simulink model "Design_qrate"  (R2017a)
settings: Solver=VariableStepAuto  StartTime=0.0  StopTime=20  RelTol=1e-3  EnableMultiTasking=on
InitFcn:
  | clear all; load('Parameters.mat');
undefined symbols (not defined in the file or in its folder): trim_control_hi
libraries: simulink x1
settings Model: Creator=Y Nie  LastModifiedBy=aelabuser
settings DataIOCC: SaveFormat=Array  SignalLoggingSaveFormat=ModelDataLogs  SaveOutput=off  SignalLogging=off  DSMLogging=off  TimeSaveName=DesignTime
settings OptimizationCC: ExpressionDepthLimit=2147483647  LifeSpan=inf
settings DebuggingCC: UnderspecifiedInitializationDetection=Classic  MergeDetectMultiDrivingBlocksExec=none  FcnCallInpInsideContextMsg=warning  StateNameClashWarn=warning  SFUnexpectedBacktrackingDiag=warning  SFNoUnconditionalDefaultTransitionDiag=warning  SFExecutionAtInitializationDiag=none
settings HardwareCC: ProdBitPerPointer=32  ProdBitPerSizeT=32  ProdBitPerPtrDiffT=32  ProdLargestAtomicFloat=None  ProdIntDivRoundTo=Undefined  ProdEndianess=Unspecified  ProdWordSize=32  ProdHWDeviceType=32-bit Generic
settings ModelReferenceCC: PropagateSignalLabelsOutOfModel=off
settings GRTTargetCC: TargetLangStandard=C89/C90 (ANSI)  GeneratePreprocessorConditionals=Disable all  CombineOutputUpdateFcns=off  GRTInterface=on
settings ConfigComp: CovMetricSettings=dw  CovHtmlReporting=on  CovSaveCumulativeToWorkspaceVar=on  CovSaveSingleToWorkspaceVar=on  CovExternalEMLEnable=off

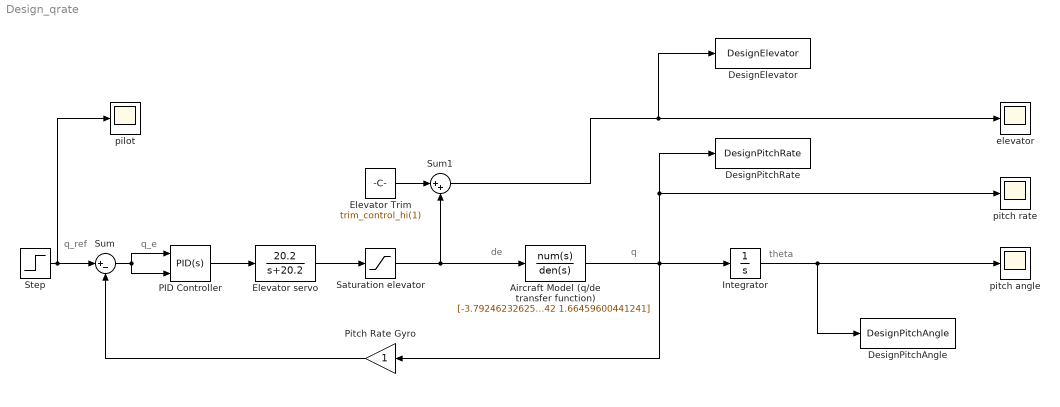
== system Design_qrate ==
  note: q_e
  note: de
  note: q
  note: theta
  note: q_ref
  Aircraft Model (q/de transfer function) : TransferFcn  Numerator=[-3.79246232625222 -2.17961147447550]  Denominator=[1 1.49753537373142 1.66459600441241]
  DesignElevator : ToWorkspace  VariableName=DesignElevator  SampleTime=-1
  DesignPitchAngle : ToWorkspace  VariableName=DesignPitchAngle  SampleTime=-1
  DesignPitchRate : ToWorkspace  VariableName=DesignPitchRate  SampleTime=-1
  Elevator Trim : Constant  Value=trim_control_hi(1)
  Elevator servo : TransferFcn  Numerator=[20.2]  Denominator=[1 20.2]
  Integrator : Integrator
  PID Controller : simulink/Continuous/PID Controller  Controller=PID  TimeDomain=Continuous-time  SampleTime=-1  IntegratorMethod=Forward Euler  FilterMethod=Forward Euler  Form=Parallel  UseFilter=on  ControllerParametersSource=internal  P=-10  I=-7  D=0  N=100  InitialConditionSource=internal  InitialConditionForIntegrator=0  InitialConditionForFilter=0  ExternalReset=either  LimitOutput=off  UpperSaturationLimit=inf  LowerSaturationLimit=-inf  LinearizeAsGain=on  AntiWindupMode=none  Kb=1  TrackingMode=off  Kt=1  PParamMin=[]  PParamMax=[]  IParamMin=[]  IParamMax=[]  DParamMin=[]  DParamMax=[]  NParamMin=[]  NParamMax=[]  KbParamMin=[]  KbParamMax=[]  KtParamMin=[]  KtParamMax=[]  POutMin=[]  POutMax=[]  IOutMin=[]  IOutMax=[]  DOutMin=[]  DOutMax=[]  NOutMin=[]  NOutMax=[]  KbOutMin=[]  KbOutMax=[]  KtOutMin=[]  KtOutMax=[]  IntegratorOutMin=[]  IntegratorOutMax=[]  FilterOutMin=[]  FilterOutMax=[]  SumOutMin=[]  SumOutMax=[]  SumI1OutMin=[]  SumI1OutMax=[]  SumI2OutMin=[]  SumI2OutMax=[]  SumI3OutMin=[]  SumI3OutMax=[]  SumDOutMin=[]  SumDOutMax=[]  SaturationOutMin=[]  SaturationOutMax=[]  IntegratorContinuousStateAttributes=''  IntegratorStateMustResolveToSignalObject=off  IntegratorRTWStateStorageClass=Auto  FilterContinuousStateAttributes=''  FilterStateMustResolveToSignalObject=off  FilterRTWStateStorageClass=Auto  DifferentiatorICPrevScaledInput=0  DifferentiatorOutMin=[]  DifferentiatorOutMax=[]  InitialConditionSetting=State (most efficient)
  Pitch Rate Gyro : Gain
  Saturation elevator : Saturate  UpperLimit=25-trim_control_hi(1)  LowerLimit=-25-trim_control_hi(1)
  Step : Step  Time=10  Before=1  After=0  SampleTime=0
  Sum : Sum  Inputs=|+-
  Sum1 : Sum  Inputs=|++
  elevator : Scope
  "pilot " : Scope
  pitch angle : Scope
  pitch rate : Scope
  wires:
  Saturation elevator/1 -> Sum1/2, Aircraft Model (q/de transfer function)/1
  Sum/1 -> PID Controller/2, PID Controller/1
  Pitch Rate Gyro/1 -> Sum/2
  PID Controller/1 -> Elevator servo/1
  Step/1 -> "pilot "/1, Sum/1
  Integrator/1 -> DesignPitchAngle/1, pitch angle/1
  Aircraft Model (q/de transfer function)/1 -> Pitch Rate Gyro/1, DesignPitchRate/1, pitch rate/1, Integrator/1
  Elevator servo/1 -> Saturation elevator/1
  Elevator Trim/1 -> Sum1/1
  Sum1/1 -> elevator/1, DesignElevator/1
